simulink model "motorFFT"  (R2020a)
settings: Solver=FixedStepAuto  StartTime=0.0  StopTime=60  FixedStep=8.33e-3  RelTol=1e-3
libraries: SignalEditorBlockLib x7, powerlib x1
settings Model: Creator=Nitesh  LastModifiedBy=DELL
settings DataIOCC: ReturnWorkspaceOutputs=off
settings DebuggingCC: UnconnectedInputMsg=none  UnconnectedOutputMsg=none  UnconnectedLineMsg=none
settings ModelReferenceCC: EnableRefExpFcnMdlSchedulingChecks=off
settings RTWCC: Description=Generic Real-Time Target
settings GRTTargetCC: RTWCAPISignals=on  RTWCAPIParams=on

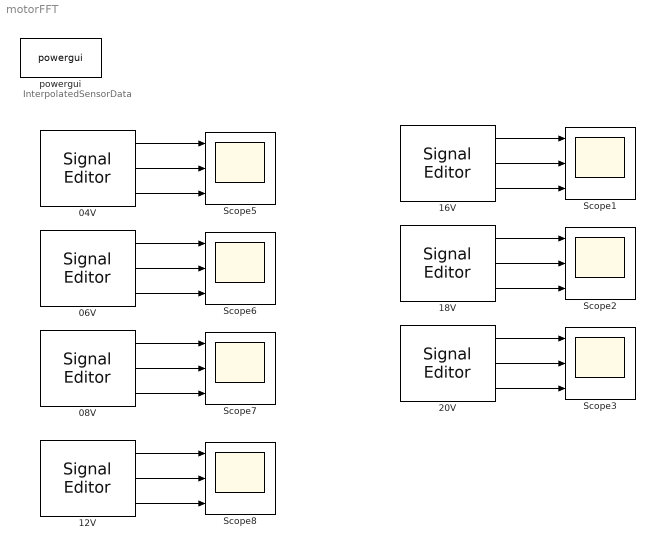
== system motorFFT ==
  note: InterpolatedSensorData
  04V : SignalEditorBlockLib/Signal Editor  FileName=_4V_scenario.mat  ActiveScenario=scenario  ActiveSignal=Ya  IsBus=off  OutputBusObjectStr=Bus: BusObject  SampleTime=0  ZeroCross=off  OutputAfterFinalValue=Setting to zero  Unit=inherit  PreserveSignalName=on
  06V : SignalEditorBlockLib/Signal Editor  FileName=_6V_scenario.mat  ActiveScenario=scenario  ActiveSignal=Za  IsBus=off  OutputBusObjectStr=Bus: BusObject  SampleTime=0  ZeroCross=off  OutputAfterFinalValue=Setting to zero  Unit=inherit  PreserveSignalName=on
  08V : SignalEditorBlockLib/Signal Editor  FileName=_8V_scenario.mat  ActiveScenario=scenario  ActiveSignal=Za  IsBus=off  OutputBusObjectStr=Bus: BusObject  SampleTime=0  ZeroCross=off  OutputAfterFinalValue=Setting to zero  Unit=inherit  PreserveSignalName=on
  12V : SignalEditorBlockLib/Signal Editor  FileName=_12V_scenario.mat  ActiveScenario=scenario  ActiveSignal=Za  IsBus=off  OutputBusObjectStr=Bus: BusObject  SampleTime=0  ZeroCross=off  OutputAfterFinalValue=Setting to zero  Unit=inherit  PreserveSignalName=on
  16V : SignalEditorBlockLib/Signal Editor  FileName=_16V_scenario.mat  ActiveScenario=scenario  ActiveSignal=Za  IsBus=off  OutputBusObjectStr=Bus: BusObject  SampleTime=0  ZeroCross=off  OutputAfterFinalValue=Setting to zero  Unit=inherit  PreserveSignalName=on
  18V : SignalEditorBlockLib/Signal Editor  FileName=_18V_scenario.mat  ActiveScenario=scenario  ActiveSignal=Za  IsBus=off  OutputBusObjectStr=Bus: BusObject  SampleTime=0  ZeroCross=off  OutputAfterFinalValue=Setting to zero  Unit=inherit  PreserveSignalName=on
  20V : SignalEditorBlockLib/Signal Editor  FileName=_20V_scenario.mat  ActiveScenario=scenario  ActiveSignal=Za  IsBus=off  OutputBusObjectStr=Bus: BusObject  SampleTime=0  ZeroCross=off  OutputAfterFinalValue=Setting to zero  Unit=inherit  PreserveSignalName=on
  Scope{1..3,5..8} (7 alike) : Scope  NumInputPorts=3
  powergui : powerlib/powergui  Priority=1  SimulationMode=Discrete  SampleTime=50e-6  frequency=60  Iterations=50  frequencyindice=60  Pbase=100e6  ErrMax=1e-4  UnitsV=kV  UnitsW=MW  buscounter=0  FunctionMessages=off  echomessages=off  EnableUseOfTLC=off  CurrentSourceSwitches=off  DisableSnubberDevices=off  DisableRonSwitches=off  DisableVfSwitches=off  DisplayEquations=off  AutomaticDiscreteSolvers=off  SolverType=Tustin/Backward Euler (TBE)  Interpol=off  ExternalGateDelay=off  methode=off  Ts=100  x0status=blocks  SPID=on  SwTol=0  HookPort=off  NonlinearTolerance=1e-4  nMaxIteration=100  ContinueOnMaxIteration=off  RestoreLinks=warning  ResistiveCurrentMeasurement=off  Frange=[0:2:500]  Ylog=off  Xlog=on  ShowGrid=off  save=off  variable=ZData  structure=smooth_20V  ZoomFFT=off  StartTime=30  cycles=10  DisplayStyle=2  fundamental=50  FreqAxis=on  MaxFrequency=500  frequencyindicesteady=1  RmsSteady=1  display=off
  wires:
  12V/1 -> Scope8/1
  08V/1 -> Scope7/1
  06V/1 -> Scope6/1
  04V/1 -> Scope5/1
  16V/1 -> Scope1/1
  18V/1 -> Scope2/1
  20V/1 -> Scope3/1
  04V/2 -> Scope5/2
  04V/3 -> Scope5/3
  06V/2 -> Scope6/2
  06V/3 -> Scope6/3
  08V/2 -> Scope7/2
  08V/3 -> Scope7/3
  12V/2 -> Scope8/2
  12V/3 -> Scope8/3
  16V/2 -> Scope1/2
  16V/3 -> Scope1/3
  18V/2 -> Scope2/2
  18V/3 -> Scope2/3
  20V/2 -> Scope3/2
  20V/3 -> Scope3/3
